simulink model "Aufgabe_10"  (Simulink 9.2)
settings: Solver=ode3  StartTime=0  StopTime=100  FixedStep=Ts  RelTol=1e-3  EnableMultiTasking=on
InitFcn:
  | Ts = 0.01; % Nicht entfernen!!!
StopFcn:
  | if Testen == 1
  | 
  | addpath('Check');
  | Aufgabe_6_Kontrolle;
  | 
  | end
libraries: dspnetwork x8, simulink x1
settings Model: Creator=Niranjan  LastModifiedBy=fleic
settings SolverCC: ZeroCrossAlgorithm=Adaptive
settings OptimizationCC: ExpressionDepthLimit=2147483647
settings DebuggingCC: SolverPrmCheckMsg=warning
settings ConfigComp: CovSFcnEnable=off

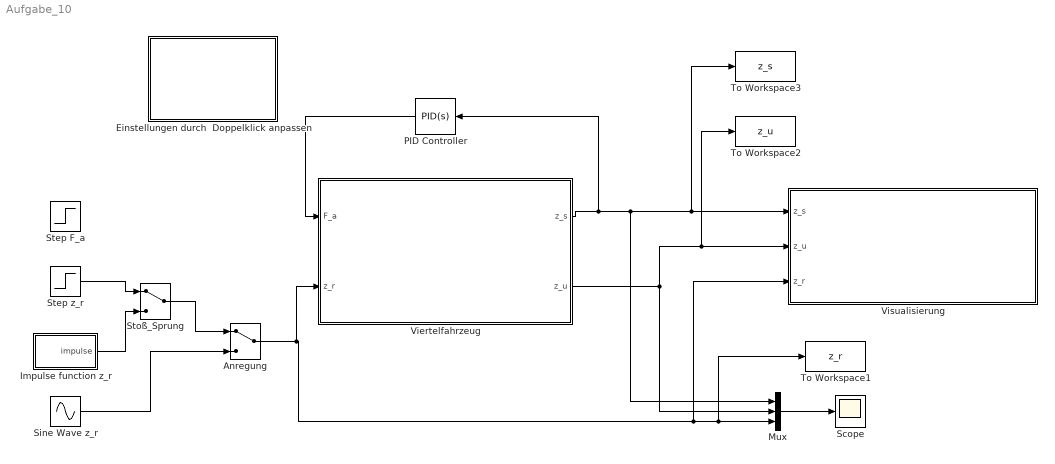
== system Aufgabe_10 ==
  Anregung : ManualSwitch
  Einstellungen durch  Doppelklick anpassen : MATLAB Function  InitFcn=tic  TreatAsAtomicUnit=on  mask{Auswahl=In Echtzeit ausführen}
      mask init:
      | maskStr = get_param(gcb,'Auswahl');
      | 
      | if strcmp(maskStr(1),'I')
      |      assignin('base','Testen',0)
      | else if strcmp(maskStr(1),'M')
      |         assignin('base','Testen',1)
      |     else
      |         assignin('base','Testen',2)
      |     end
      | end
  Impulse function z_r : Subsystem  mask{i=300, it=1}
      mask prompts: i "Verstärkungsfaktor"; it "Impulse Zeitpunkt"
  Mux : Mux  Inputs=3
  PID Controller : simulink/Continuous/PID Controller  Controller=PID  Form=Parallel  TimeDomain=Continuous-time  SampleTime=-1  IntegratorMethod=Forward Euler  FilterMethod=Forward Euler  ControllerParametersSource=internal  P=1  I=1  D=0  UseFilter=on  N=100  TunerSelectOption=Transfer Function Based (PID Tuner App)  InitialConditionSource=internal  InitialConditionForIntegrator=0  InitialConditionForFilter=0  DifferentiatorICPrevScaledInput=0  ExternalReset=none  TrackingMode=off  Kt=1  LimitOutput=off  UpperSaturationLimit=inf  LowerSaturationLimit=-inf  LinearizeAsGain=on  AntiWindupMode=none  Kb=1  POutMin=[]  POutMax=[]  IOutMin=[]  IOutMax=[]  DOutMin=[]  DOutMax=[]  NOutMin=[]  NOutMax=[]  SumOutMin=[]  SumOutMax=[]  SaturationOutMin=[]  SaturationOutMax=[]  PParamMin=[]  PParamMax=[]  IParamMin=[]  IParamMax=[]  DParamMin=[]  DParamMax=[]  NParamMin=[]  NParamMax=[]  KbParamMin=[]  KbParamMax=[]  KtParamMin=[]  KtParamMax=[]  KbOutMin=[]  KbOutMax=[]  KtOutMin=[]  KtOutMax=[]  IntegratorOutMin=[]  IntegratorOutMax=[]  FilterOutMin=[]  FilterOutMax=[]  SumI1OutMin=[]  SumI1OutMax=[]  SumI2OutMin=[]  SumI2OutMax=[]  SumI3OutMin=[]  SumI3OutMax=[]  SumI4OutMin=[]  SumI4OutMax=[]  SumDOutMin=[]  SumDOutMax=[]  DifferentiatorOutMin=[]  DifferentiatorOutMax=[]  FilterDiffOutCoefMin=[]  FilterDiffOutCoefMax=[]  ReciprocalOutMin=[]  ReciprocalOutMax=[]  SumDenOutMin=[]  SumDenOutMax=[]  SumNumOutMin=[]  SumNumOutMax=[]  DivideOutMin=[]  DivideOutMax=[]  IntegratorContinuousStateAttributes=''  IntegratorStateMustResolveToSignalObject=off  IntegratorRTWStateStorageClass=Auto  FilterContinuousStateAttributes=''  FilterStateMustResolveToSignalObject=off  FilterRTWStateStorageClass=Auto  ParallelPVariant=InternalParameters  IdealPVariant=Disabled  IVariant=InternalParameters  DVariant=InternalParameters  IntegratorVariant=Continuous  SatVariant=Disabled  AWVariant=Passthrough  PCopyVariant=Disabled  TRVariant=Disabled  FdbkBlocksVariant=Forward  IdealPFdbkVariant=Disabled  SatFdbkVariant=Disabled  DerivativeFilterVariant=ContFilter  NVariant=InternalParameters  NCopyVariant=Disabled  FilterICVariant=InternalICsFilter  IntegratorICVariant=InternalICs  ExternalResetVariant=Disabled  TRSumVariant=Passthrough  SumFdbkVariant=Disabled  SumVariant=Sum_PID
  Scope : Scope
  Sine Wave z_r : Sin  Amplitude=0.02  Frequency=2*pi  SampleTime=Ts
  Step F_a : Step  After=0  SampleTime=Ts
  Step z_r : Step  After=0.05  SampleTime=Ts
  Stoß_Sprung : ManualSwitch
  To Workspace1 : ToWorkspace  VariableName=z_r  SampleTime=Ts
  To Workspace2 : ToWorkspace  VariableName=z_u  SampleTime=Ts
  To Workspace3 : ToWorkspace  VariableName=z_s  SampleTime=Ts
  Viertelfahrzeug : Subsystem
  Visualisierung : Subsystem
      settings: OpenFcn=|
      | %!Viertelfahrzeug_Visualisierung_64bit\Viertelfahrzeug.blend.exe
      | !Viertelfahrzeug_Visualisierung_32bit\Viertelfahrzeug.blend.exe
  wires:
  Step z_r/1 -> Stoß_Sprung/1
  Impulse function z_r/1(impulse) -> Stoß_Sprung/2
  Stoß_Sprung/1 -> Anregung/1
  Sine Wave z_r/1 -> Anregung/2
  Anregung/1 -> Viertelfahrzeug/2(z_r), To Workspace1/1, Mux/3, Visualisierung/3(z_r)
  Mux/1 -> Scope/1
  Viertelfahrzeug/2(z_u) -> To Workspace2/1, Visualisierung/2(z_u), Mux/2
  Viertelfahrzeug/1(z_s) -> PID Controller/1, Mux/1, To Workspace3/1, Visualisierung/1("z_s ")
  PID Controller/1 -> Viertelfahrzeug/1(F_a)

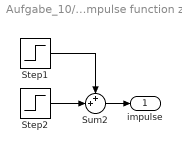
== system Aufgabe_10/Impulse function z_r ==
  Step1 : Step  Time=it  After=i  SampleTime=Ts
  Step2 : Step  Time=it+0.001  After=-i  SampleTime=Ts
  Sum2 : Sum  Inputs=++|
  impulse : Outport
  wires:
  Step2/1 -> Sum2/2
  Step1/1 -> Sum2/1
  Sum2/1 -> impulse/1

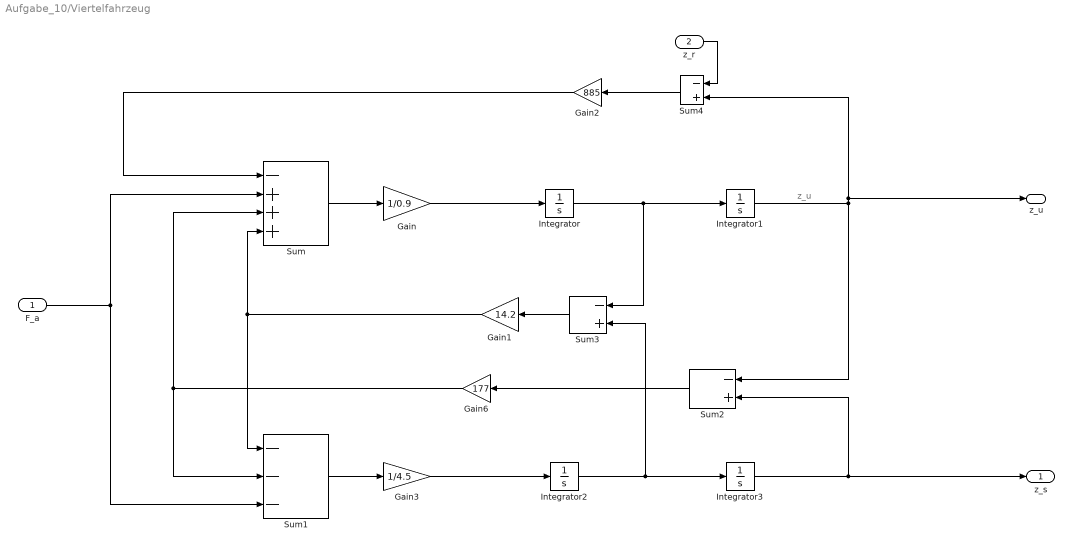
== system Aufgabe_10/Viertelfahrzeug ==
  note: z_u
  F_a : Inport  PortDimensions=1
  z_r : Inport  Port=2  PortDimensions=1
  Gain : Gain  Gain=1/0.9
  Gain1 : Gain  Gain=14.2
  Gain2 : Gain  Gain=885
  Gain3 : Gain  Gain=1/4.5
  Gain6 : Gain  Gain=177
  Integrator{,1..3} (4 alike) : Integrator
  Sum : Sum  Inputs=-+++
  Sum1 : Sum  Inputs=---
  Sum2 : Sum  Inputs=-+
  Sum3 : Sum  Inputs=-+
  Sum4 : Sum  Inputs=-+
  z_s : Outport  PortDimensions=1
  z_u : Outport  Port=2  PortDimensions=1
  wires:
  Gain6/1 -> Sum/3, Sum1/2
  Gain/1 -> Integrator/1
  Gain3/1 -> Integrator2/1
  Sum4/1 -> Gain2/1
  Integrator1/1 -> Sum4/2, z_u/1, Sum2/1
  Sum2/1 -> Gain6/1
  Gain1/1 -> Sum/4, Sum1/1
  Integrator2/1 -> Integrator3/1, Sum3/2
  Integrator/1 -> Sum3/1, Integrator1/1
  Integrator3/1 -> z_s/1, Sum2/2
  Sum/1 -> Gain/1
  Sum3/1 -> Gain1/1
  Sum1/1 -> Gain3/1
  Gain2/1 -> Sum/1
  F_a/1 -> Sum1/3, Sum/2
  z_r/1 -> Sum4/1

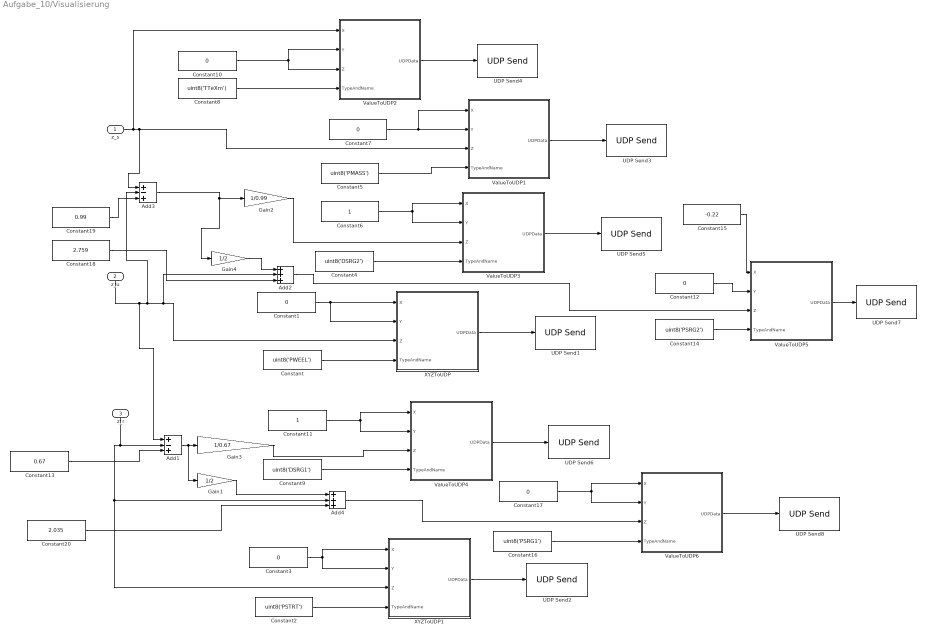
== system Aufgabe_10/Visualisierung ==
  "z_s " : Inport
  z_u : Inport  Port=2
  z_r : Inport  Port=3
  Add1 : Sum  Inputs=+-+
  Add2 : Sum  Inputs=+++
  Add3 : Sum  Inputs=+-+
  Add4 : Sum  Inputs=+++
  Constant : Constant  Value=uint8('PWEEL')
  Constant{1,3,7,10,12,17} (6 alike) : Constant  Value=0
  Constant11 : Constant
  Constant13 : Constant  Value=0.67
  Constant14 : Constant  Value=uint8('PSRG2')
  Constant15 : Constant  Value=-0.22
  Constant16 : Constant  Value=uint8('PSRG1')
  Constant18 : Constant  Value=2.759
  Constant19 : Constant  Value=0.99
  Constant2 : Constant  Value=uint8('PSTRT')
  Constant20 : Constant  Value=2.035
  Constant4 : Constant  Value=uint8('DSRG2')
  Constant5 : Constant  Value=uint8('PMASS')
  Constant6 : Constant
  Constant8 : Constant  Value=uint8('TTeXm')
  Constant9 : Constant  Value=uint8('DSRG1')
  Gain1 : Gain  Gain=1/2
  Gain2 : Gain  Gain=1/0.99
  Gain3 : Gain  Gain=1/0.67
  Gain4 : Gain  Gain=1/2
  UDP Send{1..8} (8 alike) : dspnetwork/UDP Send  remoteURL='localhost'  remotePort=9999  localURL='0.0.0.0'  localPortSource=Automatically determine  localPort=-1  sampletime=-1  blockPlatform=WINDOWS  separateLengthPort=0
      settings: SourceProductName=DSP System Toolbox  SourceProductBaseCode=DS
  ValueToUDP1 : Subsystem
  ValueToUDP2 : Subsystem
  ValueToUDP3 : Subsystem
  ValueToUDP4 : Subsystem
  ValueToUDP5 : Subsystem
  ValueToUDP6 : Subsystem
  XYZToUDP : Subsystem
  XYZToUDP1 : Subsystem
  wires:
  XYZToUDP/1(UDPData) -> UDP Send1/1
  Constant/1 -> XYZToUDP/4(TypeAndName)
  Constant1/1 -> XYZToUDP/2(Y), XYZToUDP/1(X)
  ValueToUDP1/1(UDPData) -> UDP Send3/1
  Constant5/1 -> ValueToUDP1/4(TypeAndName)
  Constant7/1 -> ValueToUDP1/1(X), ValueToUDP1/2(Y)
  ValueToUDP2/1(UDPData) -> UDP Send4/1
  Constant8/1 -> ValueToUDP2/4(TypeAndName)
  Constant10/1 -> ValueToUDP2/2(Y), ValueToUDP2/3(Z)
  "z_s "/1 -> ValueToUDP2/1(X), ValueToUDP1/3(Z), Add3/1
  XYZToUDP1/1(UDPData) -> UDP Send2/1
  Constant2/1 -> XYZToUDP1/4(TypeAndName)
  Constant3/1 -> XYZToUDP1/1(X), XYZToUDP1/2(Y)
  ValueToUDP3/1(UDPData) -> UDP Send5/1
  Constant4/1 -> ValueToUDP3/4(TypeAndName)
  Constant6/1 -> ValueToUDP3/2(Y), ValueToUDP3/1(X)
  ValueToUDP4/1(UDPData) -> UDP Send6/1
  Constant9/1 -> ValueToUDP4/4(TypeAndName)
  Constant11/1 -> ValueToUDP4/2(Y), ValueToUDP4/1(X)
  z_r/1 -> Add1/2, Add4/2, XYZToUDP1/3(Z)
  z_u/1 -> Add1/1, Add3/2, Add2/2, XYZToUDP/3(Z)
  ValueToUDP5/1(UDPData) -> UDP Send7/1
  Constant14/1 -> ValueToUDP5/4(TypeAndName)
  Constant15/1 -> ValueToUDP5/1(X)
  ValueToUDP6/1(UDPData) -> UDP Send8/1
  Constant16/1 -> ValueToUDP6/4(TypeAndName)
  Constant17/1 -> ValueToUDP6/2(Y), ValueToUDP6/1(X)
  Add1/1 -> Gain1/1, Gain3/1
  Gain3/1 -> ValueToUDP4/3(Z)
  Constant13/1 -> Add1/3
  Add4/1 -> ValueToUDP6/3(Z)
  Gain2/1 -> ValueToUDP3/3(Z)
  Constant18/1 -> Add2/3
  Gain4/1 -> Add2/1
  Add2/1 -> ValueToUDP5/3(Z)
  Constant12/1 -> ValueToUDP5/2(Y)
  Constant19/1 -> Add3/3
  Add3/1 -> Gain4/1, Gain2/1
  Constant20/1 -> Add4/3
  Gain1/1 -> Add4/1

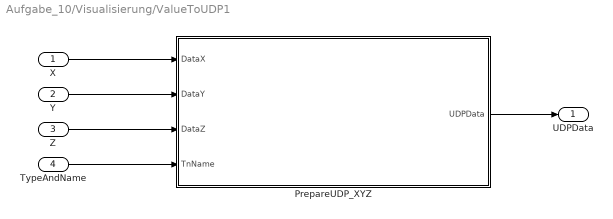
== system Aufgabe_10/Visualisierung/ValueToUDP1 ==
  X : Inport
  Y : Inport  Port=2
  Z : Inport  Port=3
  TypeAndName : Inport  Port=4
  PrepareUDP_XYZ : MATLAB Function  TreatAsAtomicUnit=on
  UDPData : Outport
  wires:
  Y/1 -> PrepareUDP_XYZ/2(DataY)
  Z/1 -> PrepareUDP_XYZ/3(DataZ)
  TypeAndName/1 -> PrepareUDP_XYZ/4(TnName)
  X/1 -> PrepareUDP_XYZ/1(DataX)
  PrepareUDP_XYZ/1(UDPData) -> UDPData/1

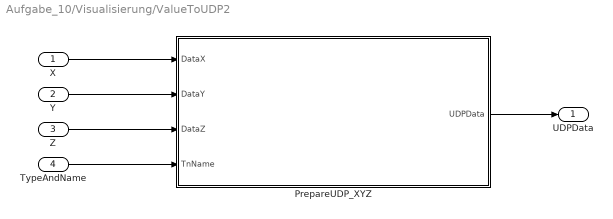
== system Aufgabe_10/Visualisierung/ValueToUDP2 ==
  X : Inport
  Y : Inport  Port=2
  Z : Inport  Port=3
  TypeAndName : Inport  Port=4
  PrepareUDP_XYZ : MATLAB Function  TreatAsAtomicUnit=on
  UDPData : Outport
  wires:
  Y/1 -> PrepareUDP_XYZ/2(DataY)
  Z/1 -> PrepareUDP_XYZ/3(DataZ)
  TypeAndName/1 -> PrepareUDP_XYZ/4(TnName)
  X/1 -> PrepareUDP_XYZ/1(DataX)
  PrepareUDP_XYZ/1(UDPData) -> UDPData/1

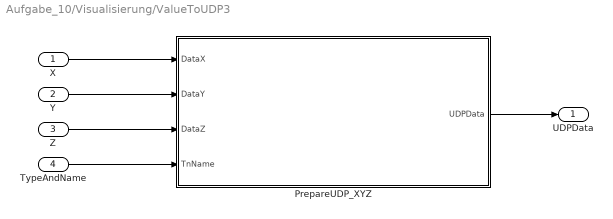
== system Aufgabe_10/Visualisierung/ValueToUDP3 ==
  X : Inport
  Y : Inport  Port=2
  Z : Inport  Port=3
  TypeAndName : Inport  Port=4
  PrepareUDP_XYZ : MATLAB Function  TreatAsAtomicUnit=on
  UDPData : Outport
  wires:
  Y/1 -> PrepareUDP_XYZ/2(DataY)
  Z/1 -> PrepareUDP_XYZ/3(DataZ)
  TypeAndName/1 -> PrepareUDP_XYZ/4(TnName)
  X/1 -> PrepareUDP_XYZ/1(DataX)
  PrepareUDP_XYZ/1(UDPData) -> UDPData/1

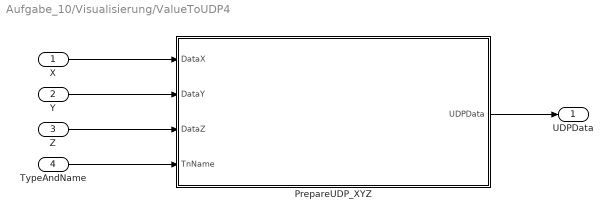
== system Aufgabe_10/Visualisierung/ValueToUDP4 ==
  X : Inport
  Y : Inport  Port=2
  Z : Inport  Port=3
  TypeAndName : Inport  Port=4
  PrepareUDP_XYZ : MATLAB Function  TreatAsAtomicUnit=on
  UDPData : Outport
  wires:
  Y/1 -> PrepareUDP_XYZ/2(DataY)
  Z/1 -> PrepareUDP_XYZ/3(DataZ)
  TypeAndName/1 -> PrepareUDP_XYZ/4(TnName)
  X/1 -> PrepareUDP_XYZ/1(DataX)
  PrepareUDP_XYZ/1(UDPData) -> UDPData/1

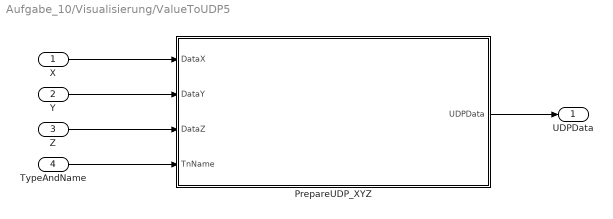
== system Aufgabe_10/Visualisierung/ValueToUDP5 ==
  X : Inport
  Y : Inport  Port=2
  Z : Inport  Port=3
  TypeAndName : Inport  Port=4
  PrepareUDP_XYZ : MATLAB Function  TreatAsAtomicUnit=on
  UDPData : Outport
  wires:
  Y/1 -> PrepareUDP_XYZ/2(DataY)
  Z/1 -> PrepareUDP_XYZ/3(DataZ)
  TypeAndName/1 -> PrepareUDP_XYZ/4(TnName)
  X/1 -> PrepareUDP_XYZ/1(DataX)
  PrepareUDP_XYZ/1(UDPData) -> UDPData/1

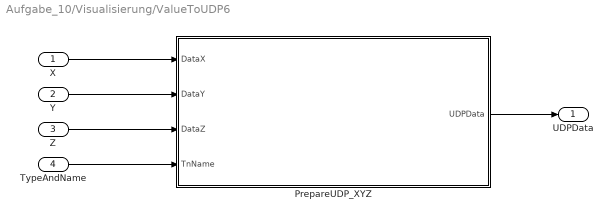
== system Aufgabe_10/Visualisierung/ValueToUDP6 ==
  X : Inport
  Y : Inport  Port=2
  Z : Inport  Port=3
  TypeAndName : Inport  Port=4
  PrepareUDP_XYZ : MATLAB Function  TreatAsAtomicUnit=on
  UDPData : Outport
  wires:
  Y/1 -> PrepareUDP_XYZ/2(DataY)
  Z/1 -> PrepareUDP_XYZ/3(DataZ)
  TypeAndName/1 -> PrepareUDP_XYZ/4(TnName)
  X/1 -> PrepareUDP_XYZ/1(DataX)
  PrepareUDP_XYZ/1(UDPData) -> UDPData/1

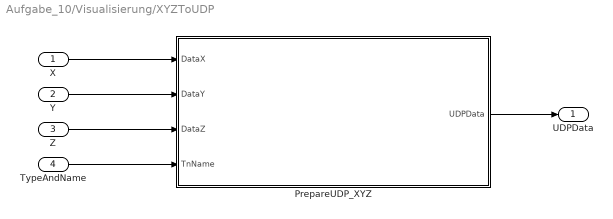
== system Aufgabe_10/Visualisierung/XYZToUDP ==
  X : Inport
  Y : Inport  Port=2
  Z : Inport  Port=3
  TypeAndName : Inport  Port=4
  PrepareUDP_XYZ : MATLAB Function  TreatAsAtomicUnit=on
  UDPData : Outport
  wires:
  Y/1 -> PrepareUDP_XYZ/2(DataY)
  Z/1 -> PrepareUDP_XYZ/3(DataZ)
  TypeAndName/1 -> PrepareUDP_XYZ/4(TnName)
  X/1 -> PrepareUDP_XYZ/1(DataX)
  PrepareUDP_XYZ/1(UDPData) -> UDPData/1

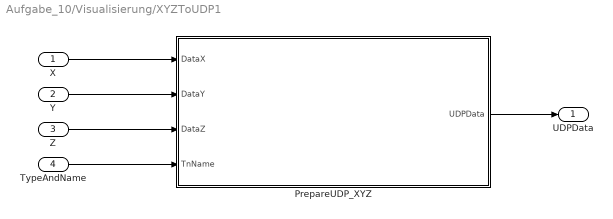
== system Aufgabe_10/Visualisierung/XYZToUDP1 ==
  X : Inport
  Y : Inport  Port=2
  Z : Inport  Port=3
  TypeAndName : Inport  Port=4
  PrepareUDP_XYZ : MATLAB Function  TreatAsAtomicUnit=on
  UDPData : Outport
  wires:
  Y/1 -> PrepareUDP_XYZ/2(DataY)
  Z/1 -> PrepareUDP_XYZ/3(DataZ)
  TypeAndName/1 -> PrepareUDP_XYZ/4(TnName)
  X/1 -> PrepareUDP_XYZ/1(DataX)
  PrepareUDP_XYZ/1(UDPData) -> UDPData/1

== matlab function Einstellungen durch Doppelklick anpassen ==
  settings: updateMethod=DISCRETE  sampleTime=0.1
function Auswahl


coder.extrinsic('tic');
coder.extrinsic('toc');
coder.extrinsic('drawnow');
coder.extrinsic('evalin');

Testen = 0;
Testen = evalin('base','Testen');

if Testen == 0

    t = 0;
    t = toc;
    while t < 0.1
    t = toc;
    drawnow;
    end
    tic;

end

== matlab function Visualisierung/ValueToUDP1/PrepareUDP_XYZ ==
  data: DataX input double; DataY input double; DataZ input double; UDPData output uint8; TnName input double
function UDPData = XYZToBlenderUdpConversion(DataX,DataY,DataZ,TnName)
tx=typecast(single(DataX),'uint8')';
ty=typecast(single(DataY),'uint8')';
tz=typecast(single(DataZ),'uint8')';
UDPData=zeros(17,1,'uint8');
UDPData=[TnName;tx;ty;tz];

== matlab function Visualisierung/ValueToUDP2/PrepareUDP_XYZ ==
  data: DataX input double; DataY input double; DataZ input double; UDPData output uint8; TnName input double
function UDPData = XYZToBlenderUdpConversion(DataX,DataY,DataZ,TnName)
tx=typecast(single(DataX),'uint8')';
ty=typecast(single(DataY),'uint8')';
tz=typecast(single(DataZ),'uint8')';
UDPData=zeros(17,1,'uint8');
UDPData=[TnName;tx;ty;tz];

== matlab function Visualisierung/ValueToUDP3/PrepareUDP_XYZ ==
  data: DataX input double; DataY input double; DataZ input double; UDPData output uint8; TnName input double
function UDPData = XYZToBlenderUdpConversion(DataX,DataY,DataZ,TnName)
tx=typecast(single(DataX),'uint8')';
ty=typecast(single(DataY),'uint8')';
tz=typecast(single(DataZ),'uint8')';
UDPData=zeros(17,1,'uint8');
UDPData=[TnName;tx;ty;tz];

== matlab function Visualisierung/ValueToUDP4/PrepareUDP_XYZ ==
  data: DataX input double; DataY input double; DataZ input double; UDPData output uint8; TnName input double
function UDPData = XYZToBlenderUdpConversion(DataX,DataY,DataZ,TnName)
tx=typecast(single(DataX),'uint8')';
ty=typecast(single(DataY),'uint8')';
tz=typecast(single(DataZ),'uint8')';
UDPData=zeros(17,1,'uint8');
UDPData=[TnName;tx;ty;tz];

== matlab function Visualisierung/ValueToUDP5/PrepareUDP_XYZ ==
  data: DataX input double; DataY input double; DataZ input double; UDPData output uint8; TnName input double
function UDPData = XYZToBlenderUdpConversion(DataX,DataY,DataZ,TnName)
tx=typecast(single(DataX),'uint8')';
ty=typecast(single(DataY),'uint8')';
tz=typecast(single(DataZ),'uint8')';
UDPData=zeros(17,1,'uint8');
UDPData=[TnName;tx;ty;tz];

== matlab function Visualisierung/ValueToUDP6/PrepareUDP_XYZ ==
  data: DataX input double; DataY input double; DataZ input double; UDPData output uint8; TnName input double
function UDPData = XYZToBlenderUdpConversion(DataX,DataY,DataZ,TnName)
tx=typecast(single(DataX),'uint8')';
ty=typecast(single(DataY),'uint8')';
tz=typecast(single(DataZ),'uint8')';
UDPData=zeros(17,1,'uint8');
UDPData=[TnName;tx;ty;tz];

== matlab function Visualisierung/XYZToUDP/PrepareUDP_XYZ ==
  data: DataX input double; DataY input double; DataZ input double; UDPData output uint8; TnName input double
function UDPData = XYZToBlenderUdpConversion(DataX,DataY,DataZ,TnName)
tx=typecast(single(DataX),'uint8')';
ty=typecast(single(DataY),'uint8')';
tz=typecast(single(DataZ),'uint8')';
UDPData=zeros(17,1,'uint8');
UDPData=[TnName;tx;ty;tz];

== matlab function Visualisierung/XYZToUDP1/PrepareUDP_XYZ ==
  data: DataX input double; DataY input double; DataZ input double; UDPData output uint8; TnName input double
function UDPData = XYZToBlenderUdpConversion(DataX,DataY,DataZ,TnName)
tx=typecast(single(DataX),'uint8')';
ty=typecast(single(DataY),'uint8')';
tz=typecast(single(DataZ),'uint8')';
UDPData=zeros(17,1,'uint8');
UDPData=[TnName;tx;ty;tz];
